simulink model "threephaseinverter1"  (R2021a)
settings: Solver=VariableStepAuto  StartTime=0.0  StopTime=10.0  RelTol=1e-3
libraries: spsIGBTDiodeLib x6, spsMultimeterLib x2, spsCurrentMeasurementLib x1, spsDCVoltageSourceLib x1, spsGroundLib x1, spsThreePhaseSeriesRLCBranchLib x1, spsVoltageMeasurementLib x1, spspowerguiLib x1
settings Model: Creator=User  LastModifiedBy=User

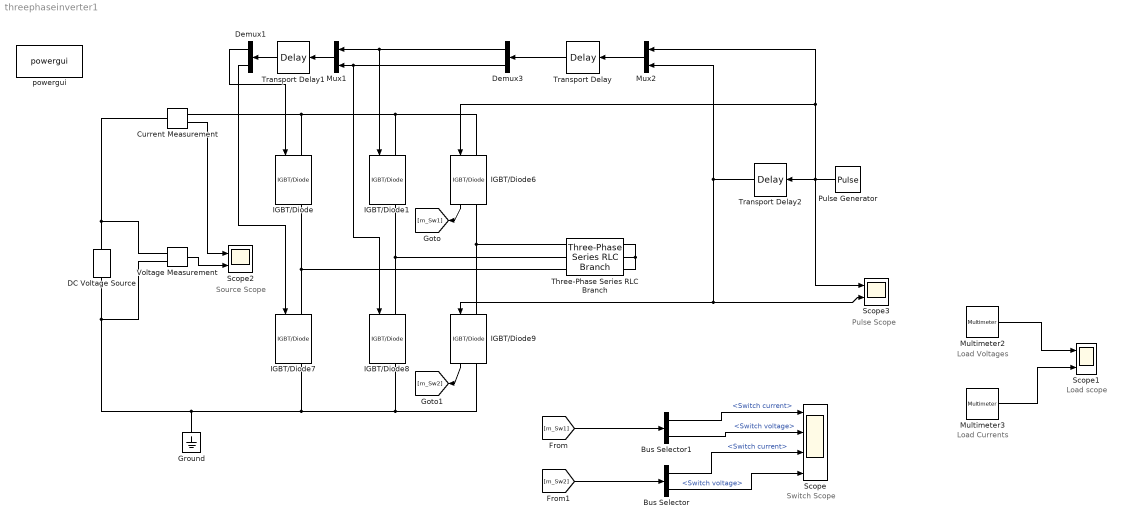
== system threephaseinverter1 ==
  note: Source Scope
  note: Switch Scope
  note: Pulse Scope
  note: Load scope
  note: Load Currents
  note: Load Voltages
  Bus Selector : BusSelector  OutputSignals=Switch current,Switch voltage
  Bus Selector1 : BusSelector  OutputSignals=Switch current,Switch voltage
  Current Measurement : spsCurrentMeasurementLib/Current Measurement  PhasorSimulation=off  OutputType=Complex  PSBequivalent=0
  DC Voltage Source : spsDCVoltageSourceLib/DC Voltage Source  Amplitude=200  Measurements=None
  Demux1 : Demux  Outputs=2
  Demux3 : Demux  Outputs=2
  Ground : spsGroundLib/Ground  LConnTagsString=a
  IGBT/Diode{,1,6..9} (6 alike) : spsIGBTDiodeLib/IGBT//Diode  Ron=1e-3  Rs=1e5  Cs=inf  Measurements=on
  Multimeter2 : spsMultimeterLib/Multimeter  PhasorSimulation=off  OutputType=Complex  sel=[1 2 3]  L=6  Gain=[1 1 1]  yselected={'Ub1: Three-Phase Series RLC Branch','Ub2: Three-Phase Series RLC Branch','Ub3: Three-Phase Series RLC Branch'};  PSBOutputType=1  PSBequivalent=0  AxesSetting=[0,0.1,-100,100]  Display=0  SavedBlockNames=-11
  Multimeter3 : spsMultimeterLib/Multimeter  PhasorSimulation=off  OutputType=Complex  sel=[4 5 6]  L=6  Gain=[1 1 1]  yselected={'Ib1: Three-Phase Series RLC Branch','Ib2: Three-Phase Series RLC Branch','Ib3: Three-Phase Series RLC Branch'};  PSBOutputType=1  PSBequivalent=0  AxesSetting=[0,0.1,-100,100]  Display=0  SavedBlockNames=-11
  Mux1 : Mux  Inputs=2
  Mux2 : Mux  Inputs=2
  Pulse Generator : DiscretePulseGenerator  PulseType=Time based  Period=0.02  PulseWidth=49.99
  Scope : Scope  NumInputPorts=4
  Scope1 : Scope  NumInputPorts=2
  Scope2 : Scope  NumInputPorts=2
  Scope3 : Scope  NumInputPorts=2
  Three-Phase Series RLC Branch : spsThreePhaseSeriesRLCBranchLib/Three-Phase Series RLC Branch  LConnTagsString=A|B|C  RConnTagsString=A|B|C  BranchType=RL  Resistance=100  Inductance=1  Capacitance=1e-6  Measurements=Branch voltages and currents
  Transport Delay : TransportDelay  DelayTime=120*0.01/180
  Transport Delay1 : TransportDelay  DelayTime=120*0.01/180
  Transport Delay2 : TransportDelay  DelayTime=0.01
  Voltage Measurement : spsVoltageMeasurementLib/Voltage Measurement  PhasorSimulation=off  OutputType=Complex  PSBequivalent=0
  powergui : spspowerguiLib/powergui  Priority=1  SimulationMode=Discrete  SampleTime=5e-5  frequency=60  Iterations=50  frequencyindice=0  Pbase=100e6  ErrMax=1e-4  UnitsV=kV  UnitsW=MW  buscounter=0  FunctionMessages=off  echomessages=off  EnableUseOfTLC=off  CurrentSourceSwitches=off  DisableSnubberDevices=off  DisableRonSwitches=off  DisableVfSwitches=off  DisplayEquations=off  AutomaticDiscreteSolvers=off  SolverType=Tustin/Backward Euler (TBE)  Interpol=off  ExternalGateDelay=off  methode=off  Ts=100  x0status=blocks  SPID=on  SwTol=0  HookPort=off  NonlinearTolerance=1e-4  nMaxIteration=100  ContinueOnMaxIteration=off  RestoreLinks=warning  ResistiveCurrentMeasurement=off  Frange=[0:2:500]  Ylog=off  Xlog=on  ShowGrid=off  save=off  variable=ZData  structure=0  ZoomFFT=off  StartTime=0.0  cycles=1  DisplayStyle=1  fundamental=60  FreqAxis=off  MaxFrequency=1000  frequencyindicesteady=1  RmsSteady=1  display=off
  wires:
  IGBT/Diode9/1 -> [m_Sw2]
  IGBT/Diode6/1 -> [m_Sw1]
  Current Measurement/1 -> Scope2/1
  Voltage Measurement/1 -> Scope2/2
  Pulse Generator/1 -> IGBT/Diode6/1, Mux2/1, Scope3/1, Transport Delay2/1
  Transport Delay2/1 -> Mux2/2, Scope3/2, IGBT/Diode9/1
  Mux2/1 -> Transport Delay/1
  Transport Delay/1 -> Demux3/1
  Demux3/1 -> IGBT/Diode1/1, Mux1/1
  Demux3/2 -> IGBT/Diode8/1, Mux1/2
  Mux1/1 -> Transport Delay1/1
  Transport Delay1/1 -> Demux1/1
  Demux1/1 -> IGBT/Diode/1
  Demux1/2 -> IGBT/Diode7/1
  [m_Sw1] -> Bus Selector1/1
  [m_Sw2] -> Bus Selector/1
  Bus Selector1/1 -> Scope/1  "<Switch current>"
  Bus Selector1/2 -> Scope/2  "<Switch voltage>"
  Bus Selector/1 -> Scope/3  "<Switch current>"
  Bus Selector/2 -> Scope/4  "<Switch voltage>"
  Multimeter2/1 -> Scope1/1
  Multimeter3/1 -> Scope1/2
  connections:
  DC Voltage Source/RConn1 -- Voltage Measurement/LConn1 -- Current Measurement/LConn1
  Current Measurement/RConn1 -- IGBT/Diode6/LConn1 -- IGBT/Diode1/LConn1 -- IGBT/Diode/LConn1
  IGBT/Diode/RConn1 -- Three-Phase Series RLC Branch/LConn3 -- IGBT/Diode7/LConn1
  IGBT/Diode1/RConn1 -- Three-Phase Series RLC Branch/LConn2 -- IGBT/Diode8/LConn1
  IGBT/Diode6/RConn1 -- Three-Phase Series RLC Branch/LConn1 -- IGBT/Diode9/LConn1
  DC Voltage Source/LConn1 -- Voltage Measurement/LConn2 -- Ground/LConn1 -- IGBT/Diode9/RConn1 -- IGBT/Diode8/RConn1 -- IGBT/Diode7/RConn1
  Three-Phase Series RLC Branch/RConn1 -- Three-Phase Series RLC Branch/RConn3 -- Three-Phase Series RLC Branch/RConn2
